simulink model "quest3_app2"  (R2015a)
settings: Solver=ode3  StartTime=0.0  StopTime=100  FixedStep=0.01  RelTol=1e-3
values from neighbouring files (symbols this model uses):
  Kd = 10    [dynamicInit.m]
  Kp = 25    [dynamicInit.m]
  L = 0.13    [dynamicInit.m]
  r = 0.1    [dynamicInit.m]
  Xfinal = -2    [dynamicInit.m]
  Yfinal = 1.5    [dynamicInit.m]
undefined symbols (not defined in the file or in its folder): F_invW_2
libraries: simulink x2
settings Model: CovModelRefEnable=off  Creator=Subodh  LastModifiedBy=Subodh
settings SolverCC: AlgebraicLoopSolver=LineSearch
settings DataIOCC: SaveFormat=Dataset
settings HardwareCC: ProdBitPerPointer=64  ProdLargestAtomicFloat=Float  ProdIntDivRoundTo=Zero  ProdEndianess=LittleEndian  ProdHWDeviceType=Specified
settings GRTTargetCC: GeneratePreprocessorConditionals=Use local settings

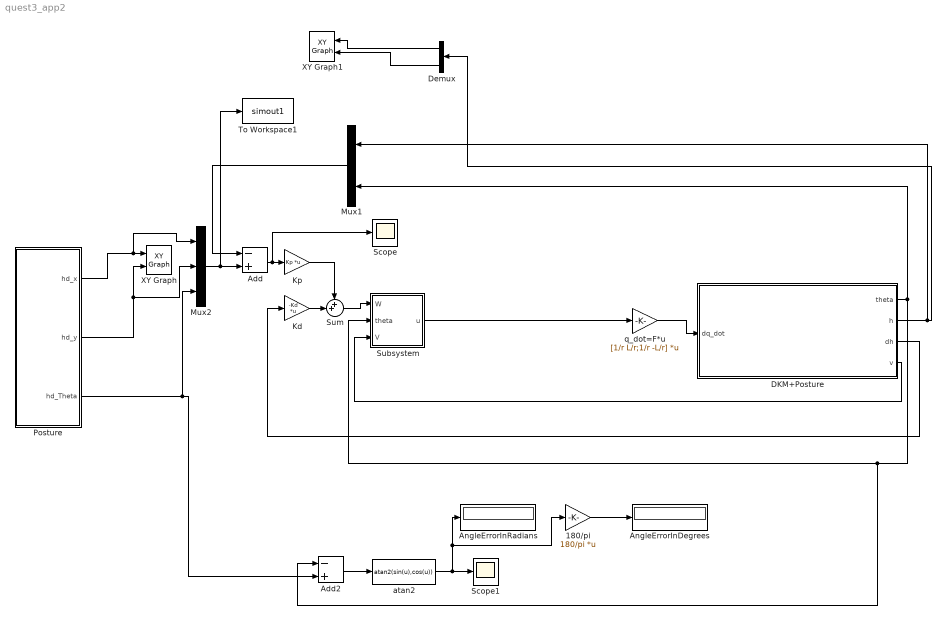
== system quest3_app2 ==
  180/pi : Gain  Gain=180/pi  Multiplication=Matrix(K*u)
  Add : Sum  Inputs=-+
  Add2 : Sum  Inputs=-+
  AngleErrorInDegrees : Display
  AngleErrorInRadians : Display
  DKM+Posture : Subsystem
  Demux : Demux  Outputs=2
  Kd : Gain  Gain=-Kd  Multiplication=Matrix(K*u)
  Kp : Gain  Gain=Kp  Multiplication=Matrix(K*u)
  Mux1 : Mux  Inputs=2
  Mux2 : Mux  Inputs=3
  Posture : Subsystem
  Scope : Scope
      settings: TimeRange=auto  MaxDataPoints=5000  SaveToWorkspace=off  SaveName=ScopeData  YMin=-0.35  YMax=0.14999  SampleTime=-1
  Scope1 : Scope
      settings: TimeRange=auto  MaxDataPoints=5000  SaveToWorkspace=off  YMin=304.4199  YMax=336.4641  SampleTime=-1
  Subsystem : Subsystem
  Sum : Sum  Inputs=++|
  To Workspace1 : ToWorkspace  VariableName=simout1  SampleTime=-1
  XY Graph : simulink/Sinks/XY Graph  xmin=-2.3  xmax=2.3  ymin=-2.3  ymax=2.3  st=-1
  XY Graph1 : simulink/Sinks/XY Graph  xmin=-2.3  xmax=2.3  ymin=-2.3  ymax=2.3  st=-1
  atan2 : Fcn  Expr=atan2(sin(u),cos(u))
  q_dot=F*u : Gain  Gain=[1/r L/r;1/r -L/r]  Multiplication=Matrix(K*u)
  wires:
  Posture/1(hd_x) -> Mux2/1, XY Graph/1
  Posture/2(hd_y) -> XY Graph/2, Mux2/2
  Mux2/1 -> To Workspace1/1, Add/2
  Add/1 -> Scope/1, Kp/1
  Kp/1 -> Sum/1
  Sum/1 -> Subsystem/1(W)
  q_dot=F*u/1 -> DKM+Posture/1(dq_dot)
  Demux/1 -> XY Graph1/1
  Demux/2 -> XY Graph1/2
  Kd/1 -> Sum/2
  DKM+Posture/3(dh) -> Kd/1
  Subsystem/1(u) -> q_dot=F*u/1
  DKM+Posture/1(theta) -> Add2/1, Subsystem/2(theta), Mux1/2
  DKM+Posture/2(h) -> Mux1/1, Demux/1
  DKM+Posture/4(v) -> Subsystem/3(V)
  Add2/1 -> atan2/1
  atan2/1 -> 180/pi/1, AngleErrorInRadians/1, Scope1/1
  180/pi/1 -> AngleErrorInDegrees/1
  Posture/3(hd_Theta) -> Add2/2, Mux2/3
  Mux1/1 -> Add/1

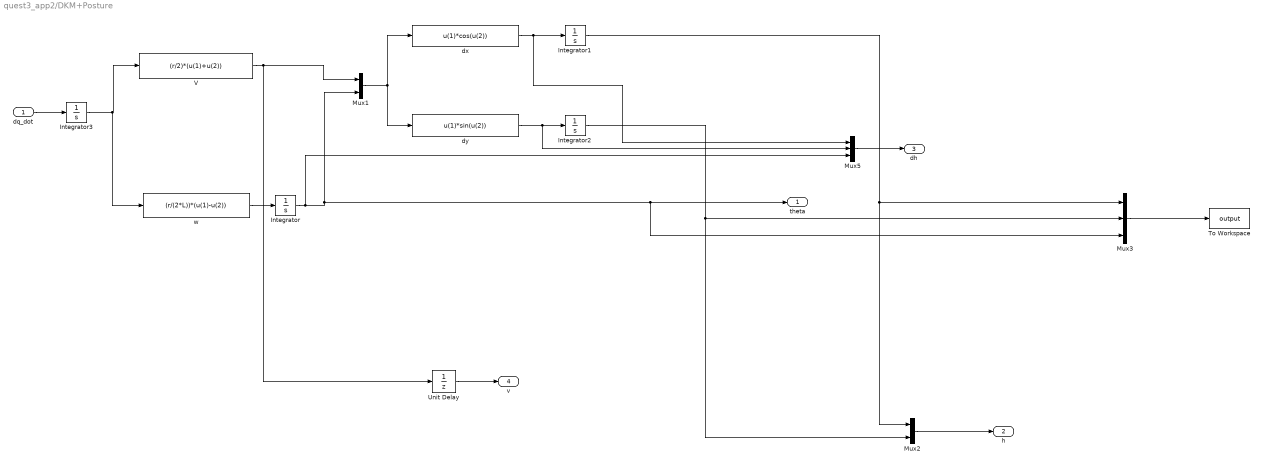
== system quest3_app2/DKM+Posture ==
  dq_dot : Inport
  Integrator : Integrator  InitialCondition=pi
  Integrator1 : Integrator  InitialCondition=2.3
  Integrator2 : Integrator
  Integrator3 : Integrator
  Mux1 : Mux  Inputs=2
  Mux2 : Mux  Inputs=2
  Mux3 : Mux  Inputs=3
  Mux5 : Mux  Inputs=3
  To Workspace : ToWorkspace  VariableName=output  SampleTime=-1
  Unit Delay : UnitDelay  SampleTime=-1
  V : Fcn  Expr=(r/2)*(u(1)+u(2))
  dx : Fcn  Expr=u(1)*cos(u(2))
  dy : Fcn  Expr=u(1)*sin(u(2))
  w : Fcn  Expr=(r/(2*L))*(u(1)-u(2))
  theta : Outport
  h : Outport  Port=2
  dh : Outport  Port=3
  v : Outport  Port=4
  wires:
  dy/1 -> Mux5/2, Integrator2/1
  Mux1/1 -> dy/1, dx/1
  dx/1 -> Mux5/1, Integrator1/1
  Mux2/1 -> h/1
  Mux5/1 -> dh/1
  Integrator1/1 -> Mux3/1, Mux2/1
  Integrator2/1 -> Mux2/2, Mux3/2
  Mux3/1 -> To Workspace/1
  V/1 -> Unit Delay/1, Mux1/1
  Integrator/1 -> Mux5/3, Mux3/3, theta/1, Mux1/2
  Unit Delay/1 -> v/1
  w/1 -> Integrator/1
  dq_dot/1 -> Integrator3/1
  Integrator3/1 -> w/1, V/1

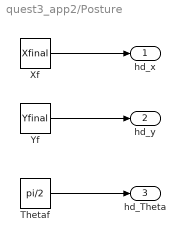
== system quest3_app2/Posture ==
  Thetaf : Constant  Value=pi/2
  Xf : Constant  Value=Xfinal
  Yf : Constant  Value=Yfinal
  hd_x : Outport
  hd_y : Outport  Port=2
  hd_Theta : Outport  Port=3
  wires:
  Xf/1 -> hd_x/1
  Yf/1 -> hd_y/1
  Thetaf/1 -> hd_Theta/1

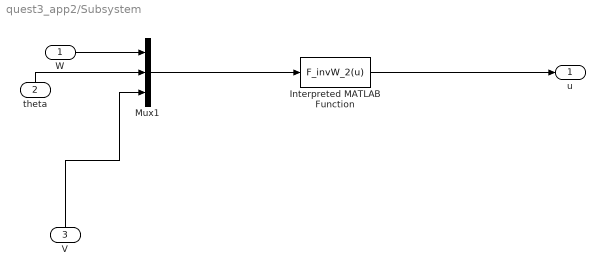
== system quest3_app2/Subsystem ==
  W : Inport
  theta : Inport  Port=2
  V : Inport  Port=3
  Interpreted MATLAB Function : MATLABFcn  MATLABFcn=F_invW_2(u)  OutputDimensions=[2 1]  OutputSignalType=real  Output1D=off
  Mux1 : Mux  Inputs=3
  u : Outport
  wires:
  theta/1 -> Mux1/2
  W/1 -> Mux1/1
  Interpreted MATLAB Function/1 -> u/1
  Mux1/1 -> Interpreted MATLAB Function/1
  V/1 -> Mux1/3
